simulink library "tcm_rebuild_voithDiwaNXT_DIWA_NXT"  (R2016a)
settings: Solver=ode1  StartTime=0.0  StopTime=10.0  FixedStep=0.01  RelTol=1e-3
undefined symbols (not defined in the file): sMP
settings Model: Creator=pethama  LastModifiedBy=mhudelm
settings DataIOCC: LimitDataPoints=on  SaveFormat=Array
settings DebuggingCC: SolverPrmCheckMsg=warning
settings HardwareCC: ProdBitPerPointer=32  ProdLargestAtomicFloat=None  ProdIntDivRoundTo=Undefined  ProdEndianess=Unspecified  ProdWordSize=32  ProdHWDeviceType=32-bit Generic
settings ModelReferenceCC: PropagateSignalLabelsOutOfModel=off
settings ConfigComp: CovSFcnEnable=off

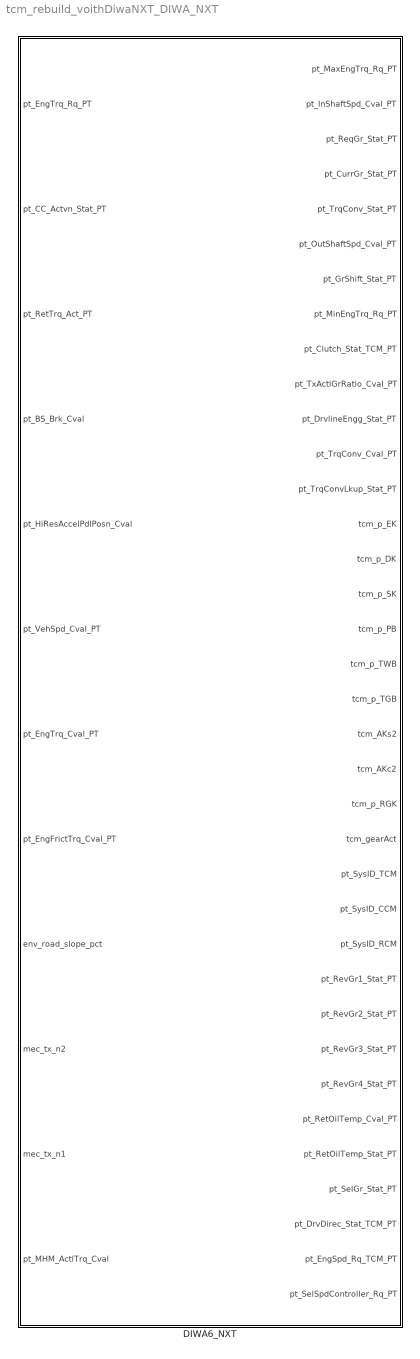
== system tcm_rebuild_voithDiwaNXT_DIWA_NXT ==
  DIWA6_NXT : Subsystem  mask{DIWA_BB_ParNames=sMP.ctrl.tcm.DIWA_BB_ParNames, DIWA_BB_ParValues=sMP.ctrl.tcm.DIWA_BB_ParValues, sVoithData=sMP.ctrl.tcm.sVoithData}
      mask prompts: sVoithData "Parameter Folder"
      mask DialogControl DescTextVar Prompt: (Add text here)

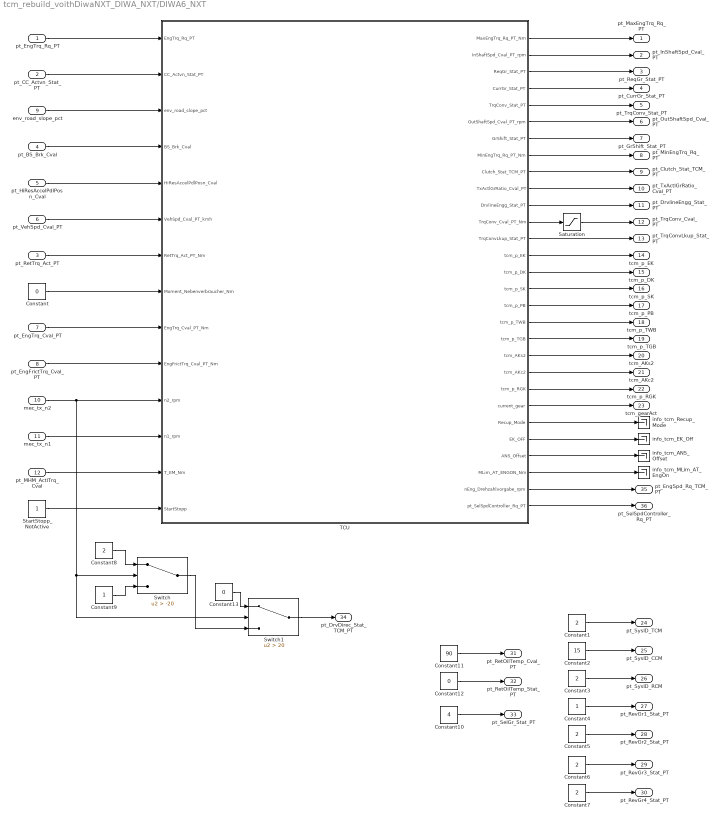
== system tcm_rebuild_voithDiwaNXT_DIWA_NXT/DIWA6_NXT ==
  pt_EngTrq_Rq_PT : Inport
  pt_CC_Actvn_Stat_PT : Inport  Port=2
  pt_RetTrq_Act_PT : Inport  Port=3
  pt_BS_Brk_Cval : Inport  Port=4
  pt_HiResAccelPdlPosn_Cval : Inport  Port=5
  pt_VehSpd_Cval_PT : Inport  Port=6
  pt_EngTrq_Cval_PT : Inport  Port=7
  pt_EngFrictTrq_Cval_PT : Inport  Port=8
  env_road_slope_pct : Inport  Port=9
  mec_tx_n2 : Inport  Port=10
  mec_tx_n1 : Inport  Port=11
  pt_MHM_ActlTrq_Cval : Inport  Port=12
  Constant : Constant  Value=0
  Constant{1,3,5..8} (6 alike) : Constant  Value=2
  Constant10 : Constant  Value=4
  Constant11 : Constant  Value=90
  Constant12 : Constant  Value=0
  Constant13 : Constant  Value=0
  Constant2 : Constant  Value=15
  Constant4 : Constant
  Constant9 : Constant
  Saturation : Saturate  UpperLimit=8107  LowerLimit=0
  StartStopp_NotActive : Constant
  Switch : Switch  Criteria=u2 > Threshold  Threshold=-20
  Switch1 : Switch  Criteria=u2 > Threshold  Threshold=20
  TCU : Subsystem
  info_tcm_ANS_Offset : Terminator
  info_tcm_EK_Off : Terminator
  info_tcm_MLim_AT_EngOn : Terminator
  info_tcm_Recup_Mode : Terminator
  pt_MaxEngTrq_Rq_PT : Outport
  pt_InShaftSpd_Cval_PT : Outport  Port=2
  pt_ReqGr_Stat_PT : Outport  Port=3
  pt_CurrGr_Stat_PT : Outport  Port=4
  pt_TrqConv_Stat_PT : Outport  Port=5
  pt_OutShaftSpd_Cval_PT : Outport  Port=6
  pt_GrShift_Stat_PT : Outport  Port=7
  pt_MinEngTrq_Rq_PT : Outport  Port=8
  pt_Clutch_Stat_TCM_PT : Outport  Port=9
  pt_TxActlGrRatio_Cval_PT : Outport  Port=10
  pt_DrvlineEngg_Stat_PT : Outport  Port=11
  pt_TrqConv_Cval_PT : Outport  Port=12
  pt_TrqConvLkup_Stat_PT : Outport  Port=13
  tcm_p_EK : Outport  Port=14
  tcm_p_DK : Outport  Port=15
  tcm_p_SK : Outport  Port=16
  tcm_p_PB : Outport  Port=17
  tcm_p_TWB : Outport  Port=18
  tcm_p_TGB : Outport  Port=19
  tcm_AKs2 : Outport  Port=20
  tcm_AKc2 : Outport  Port=21
  tcm_p_RGK : Outport  Port=22
  tcm_gearAct : Outport  Port=23
  pt_SysID_TCM : Outport  Port=24
  pt_SysID_CCM : Outport  Port=25
  pt_SysID_RCM : Outport  Port=26
  pt_RevGr1_Stat_PT : Outport  Port=27
  pt_RevGr2_Stat_PT : Outport  Port=28
  pt_RevGr3_Stat_PT : Outport  Port=29
  pt_RevGr4_Stat_PT : Outport  Port=30
  pt_RetOilTemp_Cval_PT : Outport  Port=31
  pt_RetOilTemp_Stat_PT : Outport  Port=32
  pt_SelGr_Stat_PT : Outport  Port=33
  pt_DrvDirec_Stat_TCM_PT : Outport  Port=34
  pt_EngSpd_Rq_TCM_PT : Outport  Port=35
  pt_SelSpdController_Rq_PT : Outport  Port=36
  wires:
  mec_tx_n1/1 -> TCU/12(n1_rpm)
  pt_EngFrictTrq_Cval_PT/1 -> TCU/10(EngFrictTrq_Cval_PT_Nm)
  pt_EngTrq_Cval_PT/1 -> TCU/9(EngTrq_Cval_PT_Nm)
  Constant/1 -> TCU/8(Moment_Nebenverbraucher_Nm)
  pt_VehSpd_Cval_PT/1 -> TCU/6(VehSpd_Cval_PT_kmh)
  pt_HiResAccelPdlPosn_Cval/1 -> TCU/5(HiResAccelPdlPosn_Cval)
  pt_BS_Brk_Cval/1 -> TCU/4(BS_Brk_Cval)
  pt_RetTrq_Act_PT/1 -> TCU/7(RetTrq_Act_PT_Nm)
  env_road_slope_pct/1 -> TCU/3(env_road_slope_pct)
  pt_CC_Actvn_Stat_PT/1 -> TCU/2(CC_Actvn_Stat_PT)
  pt_EngTrq_Rq_PT/1 -> TCU/1(EngTrq_Rq_PT)
  TCU/12(TrqConv_Cval_PT_Nm) -> Saturation/1
  Constant1/1 -> pt_SysID_TCM/1
  Constant3/1 -> pt_SysID_RCM/1
  Constant2/1 -> pt_SysID_CCM/1
  Constant4/1 -> pt_RevGr1_Stat_PT/1
  Constant5/1 -> pt_RevGr2_Stat_PT/1
  Constant6/1 -> pt_RevGr3_Stat_PT/1
  Constant7/1 -> pt_RevGr4_Stat_PT/1
  TCU/13(TrqConvLkup_Stat_PT) -> pt_TrqConvLkup_Stat_PT/1
  Saturation/1 -> pt_TrqConv_Cval_PT/1
  TCU/10(TxActlGrRatio_Cval_PT) -> pt_TxActlGrRatio_Cval_PT/1
  TCU/9(Clutch_Stat_TCM_PT) -> pt_Clutch_Stat_TCM_PT/1
  TCU/8(MinEngTrq_Rq_PT_Nm) -> pt_MinEngTrq_Rq_PT/1
  TCU/7(GrShift_Stat_PT) -> pt_GrShift_Stat_PT/1
  TCU/6(OutShaftSpd_Cval_PT_rpm) -> pt_OutShaftSpd_Cval_PT/1
  TCU/5(TrqConv_Stat_PT) -> pt_TrqConv_Stat_PT/1
  TCU/4(CurrGr_Stat_PT) -> pt_CurrGr_Stat_PT/1
  TCU/2(InShaftSpd_Cval_PT_rpm) -> pt_InShaftSpd_Cval_PT/1
  TCU/23(current_gear) -> tcm_gearAct/1
  TCU/19(tcm_p_TGB) -> tcm_p_TGB/1
  TCU/18(tcm_p_TWB) -> tcm_p_TWB/1
  TCU/17(tcm_p_PB) -> tcm_p_PB/1
  TCU/16(tcm_p_SK) -> tcm_p_SK/1
  TCU/15(tcm_p_DK) -> tcm_p_DK/1
  TCU/14(tcm_p_EK) -> tcm_p_EK/1
  TCU/11(DrvlineEngg_Stat_PT) -> pt_DrvlineEngg_Stat_PT/1
  Constant10/1 -> pt_SelGr_Stat_PT/1
  Constant11/1 -> pt_RetOilTemp_Cval_PT/1
  Constant12/1 -> pt_RetOilTemp_Stat_PT/1
  mec_tx_n2/1 -> TCU/11(n2_rpm), Switch1/2, Switch/2
  Switch1/1 -> pt_DrvDirec_Stat_TCM_PT/1
  Switch/1 -> Switch1/3
  Constant8/1 -> Switch/1
  Constant9/1 -> Switch/3
  Constant13/1 -> Switch1/1
  TCU/24(Recup_Mode) -> info_tcm_Recup_Mode/1
  TCU/25(EK_OFF) -> info_tcm_EK_Off/1
  TCU/26(ANS_Offset) -> info_tcm_ANS_Offset/1
  TCU/27(MLim_AT_ENGON_Nm) -> info_tcm_MLim_AT_EngOn/1
  pt_MHM_ActlTrq_Cval/1 -> TCU/13(T_EM_Nm)
  StartStopp_NotActive/1 -> TCU/14(StartStopp)
  TCU/3(ReqGr_Stat_PT) -> pt_ReqGr_Stat_PT/1
  TCU/20(tcm_AKs2) -> tcm_AKs2/1
  TCU/21(tcm_AKc2) -> tcm_AKc2/1
  TCU/22(tcm_p_RGK) -> tcm_p_RGK/1
  TCU/28("nEng_Drehzahlvorgabe_rpm ") -> pt_EngSpd_Rq_TCM_PT/1
  TCU/1(MaxEngTrq_Rq_PT_Nm) -> pt_MaxEngTrq_Rq_PT/1
  TCU/29(pt_SelSpdController_Rq_PT) -> pt_SelSpdController_Rq_PT/1

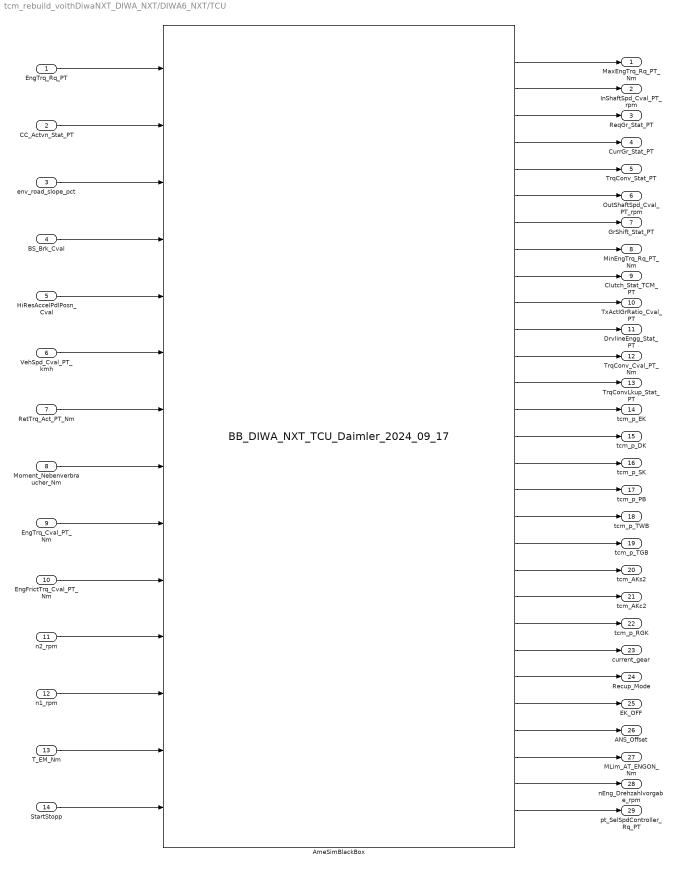
== system tcm_rebuild_voithDiwaNXT_DIWA_NXT/DIWA6_NXT/TCU ==
  EngTrq_Rq_PT : Inport
  CC_Actvn_Stat_PT : Inport  Port=2
  env_road_slope_pct : Inport  Port=3
  BS_Brk_Cval : Inport  Port=4
  HiResAccelPdlPosn_Cval : Inport  Port=5
  VehSpd_Cval_PT_kmh : Inport  Port=6
  RetTrq_Act_PT_Nm : Inport  Port=7
  Moment_Nebenverbraucher_Nm : Inport  Port=8
  EngTrq_Cval_PT_Nm : Inport  Port=9
  EngFrictTrq_Cval_PT_Nm : Inport  Port=10
  n2_rpm : Inport  Port=11
  n1_rpm : Inport  Port=12
  T_EM_Nm : Inport  Port=13
  StartStopp : Inport  Port=14
  AmeSimBlackBox : S-Function  FunctionName=BB_DIWA_NXT_TCU_Daimler_2024_09_17  Parameters=[1 0.01],DIWA_BB_ParNames,DIWA_BB_ParValues  SFunctionDeploymentMode=off  EnableBusSupport=off
      mask Display: disp('Simcenter Amesim black-box:\nBB_DIWA_NXT_TCU_Daimler_2024_09_17');port_label('input',1,'EngTrq_Rq_PT_Nm');port_label('input',2,'CC_Actvn_Stat_PT');port_label('input',3,'Streckenneigung_pc');port_label('input',4,'BS_Brk_Cval');port_label('input',5,'HiResAccelPdlPosn_Cval');port_label('input',6,'VehSpd_Cval_PT_kmh');port_label('input',7,'RetTrq_Act_PT_Nm');port_label('input',8,'Moment_Nebenverbraucher_Nm');port_label('input',9,'EngTrq_Cval_PT_Nm');port_label('input',10,'EngFrictTrq_Cval_PT_Nm');port_label('input',11,'n2_rpm');port_label('input',12,'n1_rpm');port_label('input',13,'T_EM_Nm');port_label('input',14,'StartStop');port_label('output',1,'MaxEngTrq_Rq_PT_Nm');port_label('output',2,'InShaftSp_Cval_PT_rpm');port_label('output',3,'ReqGr_Stat_PT');port_label('output',4,'CurrGr_Stat_PT');port_label('output',5,'TrqConv_Stat_PT');port_label('output',6,'OutShaftSpd_Cval_PT_rpm');port_label('output',7,'GrShift_Stat_PT');port_label('output',8,'MinEngTrq_Rq_PT_Nm');port_label('output',9,'Clutch_Stat_TCM_PT');port_label('output',10,'TxAtlGrRatio_Cval_PT');port_label('output',11,'DrvlineEngg_Stat_PT');port_label('output',12,'TrqConv_Cval_PT_Nm');port_label('output',13,'TrqConvLkup_Stat_PT');port_label('output',14,'EK_');port_label('output',15,'DK_');port_label('output',16,'SK_');port_label('output',17,'PB_');port_label('output',18,'TWB_');port_label('output',19,'TGB_');port_label('output',20,'Direktgangklaue_AKs2_');port_label('output',21,'Schnellgangklaue_AKc2_');port_label('output',22,'RGK_');port_label('output',23,'current_gear_');port_label('output',24,'Recup_Mode_');port_label('output',25,'EK_OFF_');port_label('output',26,'ANS_Offset_');port_label('output',27,'MLim_AT_ENGON_Nm');port_label('output',28,'nEng_Drehzahlvorgabe_rpm');port_label('output',29,'pt_SelSpdController_Rq_PT');
  MaxEngTrq_Rq_PT_Nm : Outport
  InShaftSpd_Cval_PT_rpm : Outport  Port=2
  ReqGr_Stat_PT : Outport  Port=3
  CurrGr_Stat_PT : Outport  Port=4
  TrqConv_Stat_PT : Outport  Port=5
  OutShaftSpd_Cval_PT_rpm : Outport  Port=6
  GrShift_Stat_PT : Outport  Port=7
  MinEngTrq_Rq_PT_Nm : Outport  Port=8
  Clutch_Stat_TCM_PT : Outport  Port=9
  TxActlGrRatio_Cval_PT : Outport  Port=10
  DrvlineEngg_Stat_PT : Outport  Port=11
  TrqConv_Cval_PT_Nm : Outport  Port=12
  TrqConvLkup_Stat_PT : Outport  Port=13
  tcm_p_EK : Outport  Port=14
  tcm_p_DK : Outport  Port=15
  tcm_p_SK : Outport  Port=16
  tcm_p_PB : Outport  Port=17
  tcm_p_TWB : Outport  Port=18
  tcm_p_TGB : Outport  Port=19
  tcm_AKs2 : Outport  Port=20
  tcm_AKc2 : Outport  Port=21
  tcm_p_RGK : Outport  Port=22
  current_gear : Outport  Port=23
  Recup_Mode : Outport  Port=24
  EK_OFF : Outport  Port=25
  ANS_Offset : Outport  Port=26
  MLim_AT_ENGON_Nm : Outport  Port=27
  "nEng_Drehzahlvorgabe_rpm " : Outport  Port=28
  pt_SelSpdController_Rq_PT : Outport  Port=29
  wires:
  AmeSimBlackBox/15 -> tcm_p_DK/1
  AmeSimBlackBox/16 -> tcm_p_SK/1
  AmeSimBlackBox/17 -> tcm_p_PB/1
  AmeSimBlackBox/18 -> tcm_p_TWB/1
  EngTrq_Rq_PT/1 -> AmeSimBlackBox/1
  AmeSimBlackBox/1 -> MaxEngTrq_Rq_PT_Nm/1
  AmeSimBlackBox/2 -> InShaftSpd_Cval_PT_rpm/1
  CC_Actvn_Stat_PT/1 -> AmeSimBlackBox/2
  AmeSimBlackBox/5 -> TrqConv_Stat_PT/1
  env_road_slope_pct/1 -> AmeSimBlackBox/3
  AmeSimBlackBox/6 -> OutShaftSpd_Cval_PT_rpm/1
  AmeSimBlackBox/7 -> GrShift_Stat_PT/1
  AmeSimBlackBox/8 -> MinEngTrq_Rq_PT_Nm/1
  AmeSimBlackBox/9 -> Clutch_Stat_TCM_PT/1
  AmeSimBlackBox/11 -> DrvlineEngg_Stat_PT/1
  EngTrq_Cval_PT_Nm/1 -> AmeSimBlackBox/9
  AmeSimBlackBox/13 -> TrqConvLkup_Stat_PT/1
  EngFrictTrq_Cval_PT_Nm/1 -> AmeSimBlackBox/10
  AmeSimBlackBox/14 -> tcm_p_EK/1
  n2_rpm/1 -> AmeSimBlackBox/11
  n1_rpm/1 -> AmeSimBlackBox/12
  AmeSimBlackBox/23 -> current_gear/1
  Moment_Nebenverbraucher_Nm/1 -> AmeSimBlackBox/8
  T_EM_Nm/1 -> AmeSimBlackBox/13
  StartStopp/1 -> AmeSimBlackBox/14
  AmeSimBlackBox/24 -> Recup_Mode/1
  AmeSimBlackBox/25 -> EK_OFF/1
  AmeSimBlackBox/26 -> ANS_Offset/1
  BS_Brk_Cval/1 -> AmeSimBlackBox/4
  RetTrq_Act_PT_Nm/1 -> AmeSimBlackBox/7
  VehSpd_Cval_PT_kmh/1 -> AmeSimBlackBox/6
  HiResAccelPdlPosn_Cval/1 -> AmeSimBlackBox/5
  AmeSimBlackBox/4 -> CurrGr_Stat_PT/1
  AmeSimBlackBox/27 -> MLim_AT_ENGON_Nm/1
  AmeSimBlackBox/10 -> TxActlGrRatio_Cval_PT/1
  AmeSimBlackBox/12 -> TrqConv_Cval_PT_Nm/1
  AmeSimBlackBox/19 -> tcm_p_TGB/1
  AmeSimBlackBox/3 -> ReqGr_Stat_PT/1
  AmeSimBlackBox/20 -> tcm_AKs2/1
  AmeSimBlackBox/21 -> tcm_AKc2/1
  AmeSimBlackBox/22 -> tcm_p_RGK/1
  AmeSimBlackBox/28 -> "nEng_Drehzahlvorgabe_rpm "/1
  AmeSimBlackBox/29 -> pt_SelSpdController_Rq_PT/1
